simulink model "Prj1CDig"  (R2022b)
settings: Solver=ode45  StartTime=0.0  StopTime=3000  RelTol=1e-6  EnableMultiTasking=on
values from neighbouring files (symbols this model uses):
  A = (Tz-Tp1)/(Tp2-Tp1)    (= 0.157044591698)    [Prj1CDig_m.m]
  B = 1 - A    (= 0.842955408302)    [Prj1CDig_m.m]
  I = -(P*Z-P)/Tc    (= 0.029088)    [Prj1CDig_m.m]
  Kp = 0.8864/256.0    (= 0.0034625)    [Prj1CDig_m.m]
  P = 0.909    [Prj1CDig_m.m]
  PO = 60    [Prj1CDig_m.m]
  Ta = 27    [Prj1CDig_m.m]
  Td = 5    [Prj1CDig_m.m]
  Tp1 = 323.16    [Prj1CDig_m.m]
  Tp2 = 37.636    [Prj1CDig_m.m]
  Ts = 1    [Prj1CDig_m.m]
  w0 = 0.09817477042468    (= 0.0981747704247)    [Prj1CDig_m.m]
settings Model: Creator=Adolfo  LastModifiedBy=adolfo
settings SolverCC: ZeroCrossControl=DisableAll  AlgebraicLoopSolver=TrustRegion
settings DataIOCC: LimitDataPoints=on  MaxDataPoints=25000  SaveFormat=Array  SignalLoggingSaveFormat=ModelDataLogs  ReturnWorkspaceOutputs=off
settings OptimizationCC: BlockReduction=off  BooleanDataType=off  ExpressionDepthLimit=2147483647  InitFltsAndDblsToZero=on  LifeSpan=inf
settings DebuggingCC: SaveWithParameterizedLinksMsg=none  UnderspecifiedInitializationDetection=Classic  MergeDetectMultiDrivingBlocksExec=none  SignalResolutionControl=TryResolveAllWithWarning  MultiTaskDSMMsg=warning  MultiTaskCondExecSysMsg=none  FcnCallInpInsideContextMsg=warning  UnconnectedInputMsg=warning  UnconnectedOutputMsg=warning  UnconnectedLineMsg=warning  StateNameClashWarn=warning  SFUnexpectedBacktrackingDiag=warning  SFNoUnconditionalDefaultTransitionDiag=warning  SFExecutionAtInitializationDiag=none  SFMachineParentedDataDiag=warning  ArithmeticOperatorsInVariantConditions=warning
settings HardwareCC: ProdBitPerPointer=32  ProdBitPerSizeT=32  ProdBitPerPtrDiffT=32  ProdLargestAtomicFloat=None  ProdIntDivRoundTo=Undefined  ProdEndianess=Unspecified  ProdWordSize=32  ProdHWDeviceType=32-bit Generic  TargetUnknown=on
settings ModelReferenceCC: PropagateSignalLabelsOutOfModel=off
settings SFSimCC: SimUseLocalCustomCode=off  CustomCodeUndefinedFunction=UseInterfaceOnly
settings RTWCC: RTWUseLocalCustomCode=off
settings CodeAppCC: StateflowObjectComments=on
settings GRTTargetCC: TargetFcnLib=ansi_tfl_tmw.mat  TargetLangStandard=C89/C90 (ANSI)  CombineOutputUpdateFcns=off  GRTInterface=on
settings ConfigComp: CovMetricSettings=dw  CovSaveCumulativeToWorkspaceVar=on  CovSaveSingleToWorkspaceVar=on

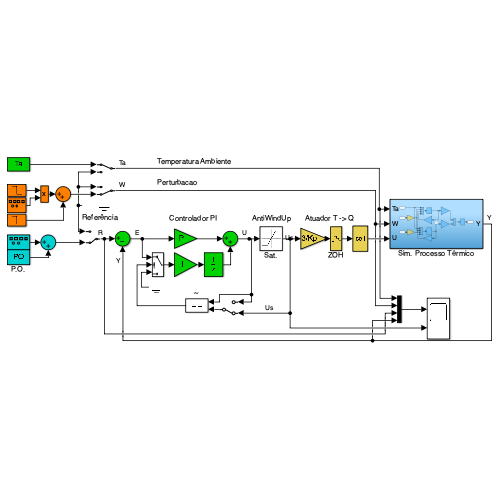
[thumbnail: Simulink's stored preview of the top-level diagram]
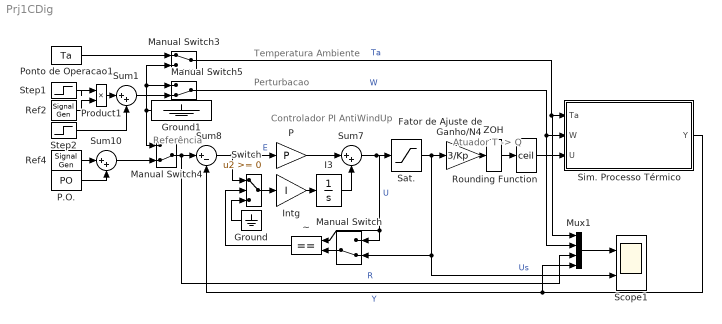
== system Prj1CDig ==
  note: Temperatura Ambiente
  note: Atuador T -> Q
  note: Referência
  note: Controlador PI AntiWindUp
  note: Perturbacao
  Fator de Ajuste de Ganho/N4 : Gain  Gain=3/Kp  SaturateOnIntegerOverflow=on  OutDataTypeStr=Inherit: Same as input  ParamDataTypeStr=Inherit: Same as input
  Ground : Ground
  Ground1 : Ground
  I3 : Integrator
  Intg : Gain  Gain=I
  Manual Switch : ManualSwitch  CurrentSetting=0
  Manual Switch3 : ManualSwitch
  Manual Switch4 : ManualSwitch  CurrentSetting=0
  Manual Switch5 : ManualSwitch  CurrentSetting=0
  Mux1 : Mux
  P : Gain  Gain=P
  P.O. : Constant  Value=PO
  Ponto de Operacao1 : Constant  Value=Ta
  Product1 : Product  RndMeth=Zero
  Ref2 : SignalGenerator  Frequency=w0  Units=rad/sec
  Ref4 : SignalGenerator  WaveForm=square  Amplitude=5  Frequency=.00125
  Rounding Function : Rounding  Operator=ceil
  Sat. : Saturate  UpperLimit=12  LowerLimit=0
  Scope1 : Scope  NumInputPorts=2
  Sim. Processo Térmico : Subsystem
  Step1 : Step  Time=2200  After=-5  SampleTime=0
  Step2 : Step  Time=1100  After=-5  SampleTime=0
  Sum1 : Sum  Inputs=|++
  Sum10 : Sum  Inputs=|++
  Sum7 : Sum  Inputs=|++
  Sum8 : Sum  Inputs=|+-
  Switch : Switch  SaturateOnIntegerOverflow=off  InputSameDT=off
  ZOH : ZeroOrderHold  SampleTime=Ts
  ~ : RelationalOperator  Operator===  OutDataTypeStr=boolean  InputSameDT=off
  wires:
  Sat./1 -> Manual Switch/2, Scope1/2, Fator de Ajuste de Ganho/N4/1  "Us"
  P.O./1 -> Sum10/2
  Sum7/1 -> ~/1, Manual Switch/1, Sat./1  "U"
  Ref4/1 -> Sum10/1
  ZOH/1 -> Rounding Function/1
  Intg/1 -> I3/1
  Switch/1 -> Intg/1
  P/1 -> Sum7/1
  Ground/1 -> Switch/3
  I3/1 -> Sum7/2
  Sum8/1 -> Switch/1, P/1  "E"
  Rounding Function/1 -> Sim. Processo Térmico/3(U)
  Fator de Ajuste de Ganho/N4/1 -> ZOH/1
  ~/1 -> Switch/2
  Manual Switch5/1 -> Mux1/2, Sim. Processo Térmico/2(W)  "W"
  Manual Switch/1 -> ~/2
  Sim. Processo Térmico/1(Y) -> Mux1/4, Sum8/2  "Y"
  Manual Switch3/1 -> Mux1/1, Sim. Processo Térmico/1(Ta)  "Ta"
  Ground1/1 -> Manual Switch3/2, Manual Switch5/1, Manual Switch4/1
  Manual Switch4/1 -> Mux1/3, Sum8/1  "R"
  Step1/1 -> Product1/1
  Ref2/1 -> Product1/2
  Sum1/1 -> Manual Switch5/2
  Ponto de Operacao1/1 -> Manual Switch3/1
  Sum10/1 -> Manual Switch4/2
  Mux1/1 -> Scope1/1
  Step2/1 -> Sum1/2
  Product1/1 -> Sum1/1

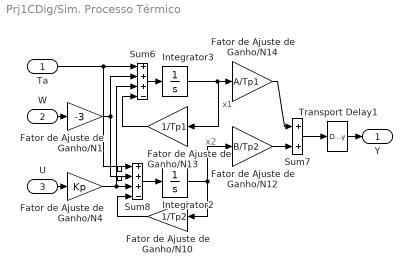
== system Prj1CDig/Sim. Processo Térmico ==
  note: x2
  Ta : Inport
  W : Inport  Port=2
  U : Inport  Port=3
  Fator de Ajuste de Ganho/N1 : Gain  Gain=-3  SaturateOnIntegerOverflow=on  OutDataTypeStr=Inherit: Same as input  ParamDataTypeStr=Inherit: Same as input
  Fator de Ajuste de Ganho/N10 : Gain  Gain=1/Tp2  SaturateOnIntegerOverflow=on  OutDataTypeStr=Inherit: Same as input  ParamDataTypeStr=Inherit: Same as input
  Fator de Ajuste de Ganho/N12 : Gain  Gain=B/Tp2  SaturateOnIntegerOverflow=on  OutDataTypeStr=Inherit: Same as input  ParamDataTypeStr=Inherit: Same as input
  Fator de Ajuste de Ganho/N13 : Gain  Gain=1/Tp1  SaturateOnIntegerOverflow=on  OutDataTypeStr=Inherit: Same as input  ParamDataTypeStr=Inherit: Same as input
  Fator de Ajuste de Ganho/N14 : Gain  Gain=A/Tp1  SaturateOnIntegerOverflow=on  OutDataTypeStr=Inherit: Same as input  ParamDataTypeStr=Inherit: Same as input
  Fator de Ajuste de Ganho/N4 : Gain  Gain=Kp  SaturateOnIntegerOverflow=on  OutDataTypeStr=Inherit: Same as input  ParamDataTypeStr=Inherit: Same as input
  Integrator2 : Integrator  InitialCondition=Ta*Tp2
  Integrator3 : Integrator  InitialCondition=Ta*Tp1
  Sum6 : Sum  Inputs=+++-
  Sum7 : Sum  InputSameDT=on  SaturateOnIntegerOverflow=on  OutDataTypeStr=Inherit: Same as first input
  Sum8 : Sum  Inputs=+++-
  Transport Delay1 : TransportDelay  DelayTime=Td  InitialOutput=Ta  PadeOrder=2
  Y : Outport
  wires:
  Sum7/1 -> Transport Delay1/1
  Fator de Ajuste de Ganho/N12/1 -> Sum7/2
  Fator de Ajuste de Ganho/N13/1 -> Sum6/4
  Sum8/1 -> Integrator2/1
  Sum6/1 -> Integrator3/1
  Fator de Ajuste de Ganho/N10/1 -> Sum8/4
  U/1 -> Fator de Ajuste de Ganho/N4/1
  Fator de Ajuste de Ganho/N14/1 -> Sum7/1
  Integrator3/1 -> Fator de Ajuste de Ganho/N14/1, Fator de Ajuste de Ganho/N13/1  "x1"
  Integrator2/1 -> Fator de Ajuste de Ganho/N12/1, Fator de Ajuste de Ganho/N10/1
  Ta/1 -> Sum6/1, Sum8/1
  W/1 -> Fator de Ajuste de Ganho/N1/1
  Fator de Ajuste de Ganho/N4/1 -> Sum8/3, Sum6/3
  Transport Delay1/1 -> Y/1
  Fator de Ajuste de Ganho/N1/1 -> Sum6/2, Sum8/2
